simulink model "test_onoff_button_wrongpressionbehavior"  (R2022b)
settings: Solver=FixedStepAuto  StartTime=0.0  StopTime=240  FixedStep=0.1  RelTol=1e-3
settings Model: Creator=alewi  LastModifiedBy=cristian
settings ConfigComp: CovEnable=on  RecordCoverage=on  CovModelRefEnable=on

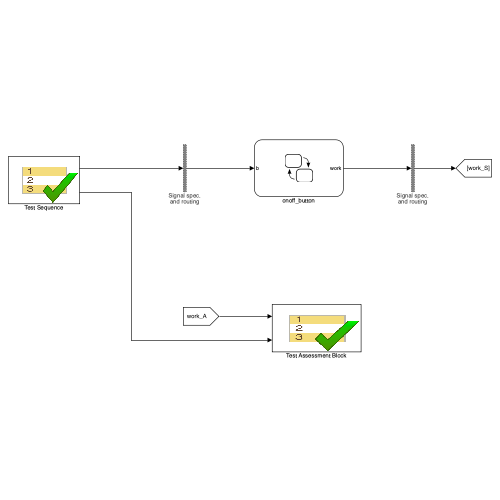
[thumbnail: Simulink's stored preview of the top-level diagram]
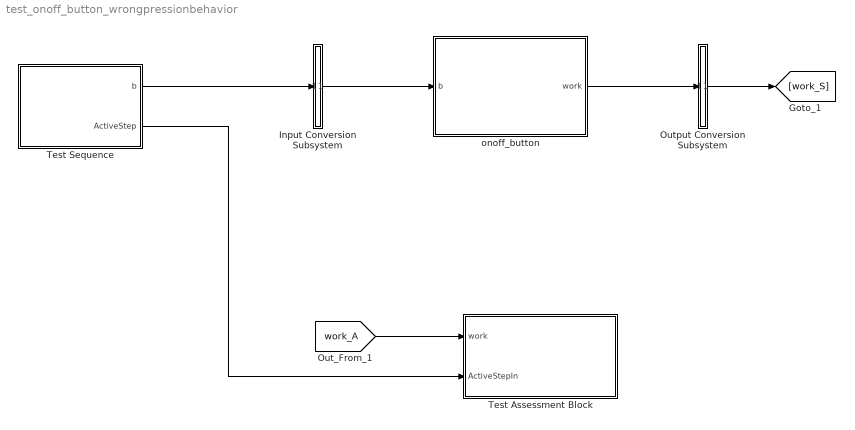
== system test_onoff_button_wrongpressionbehavior ==
  Input Conversion Subsystem : Subsystem  Tag=__SLT_ICS__  Description=|
      | Signal spec.
      | and routing
      settings: AttributesFormatString=%<Description>
  Output Conversion Subsystem : Subsystem  Tag=__SLT_OCS__  Description=|
      | Signal spec.
      | and routing
      settings: AttributesFormatString=%<Description>
  Test Assessment Block : Test Sequence  Tag=__SLT_ASMT__  TreatAsAtomicUnit=on
  Test Sequence : Test Sequence  TreatAsAtomicUnit=on
  onoff_button : Stateflow chart  TreatAsAtomicUnit=on
  wires:
  Output Conversion Subsystem/1(Outport_1) -> [work_S]
  Input Conversion Subsystem/1(Outport_1) -> onoff_button/1(b)
  onoff_button/1(work) -> Output Conversion Subsystem/1(Inport_1)
  Test Sequence/1(b) -> Input Conversion Subsystem/1(Inport_1)
  Test Sequence/2(ActiveStep) -> Test Assessment Block/2(ActiveStepIn)
  [work_A] -> Test Assessment Block/1(work)

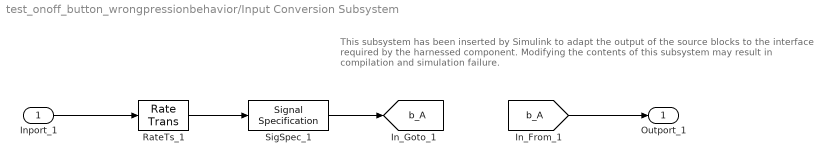
== system test_onoff_button_wrongpressionbehavior/Input Conversion Subsystem ==
  note: This subsystem has been inserted by Simulink to adapt the output of the source blocks to the interface required by the harnessed component.
      |  Modifying the contents of this subsystem may result in compilation and simulation failure.
  Inport_1 : Inport
  RateTs_1 : RateTransition  OutPortSampleTime=[-1, 0]
  SigSpec_1 : SignalSpecification  OutDataTypeStr=boolean  Dimensions=[1]  SampleTime=[-1, 0]
  Outport_1 : Outport
  tag scope: b_A=global
  wires:
  [b_A] -> Outport_1/1
  SigSpec_1/1 -> [b_A]
  RateTs_1/1 -> SigSpec_1/1
  Inport_1/1 -> RateTs_1/1

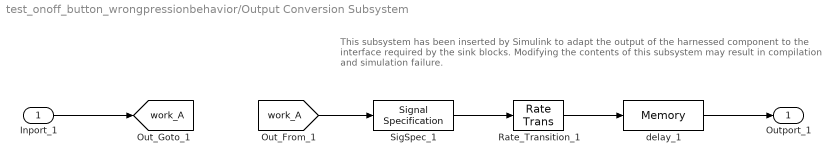
== system test_onoff_button_wrongpressionbehavior/Output Conversion Subsystem ==
  note: This subsystem has been inserted by Simulink to adapt the output of the harnessed component to the interface required by the sink blocks.
      |  Modifying the contents of this subsystem may result in compilation and simulation failure.
  Inport_1 : Inport
  Rate_Transition_1 : RateTransition  OutPortSampleTimeOpt=Inherit
  SigSpec_1 : SignalSpecification  OutDataTypeStr=boolean  Dimensions=[1]
  delay_1 : Memory
  Outport_1 : Outport
  tag scope: work_A=global
  wires:
  Inport_1/1 -> [work_A]
  [work_A] -> SigSpec_1/1
  SigSpec_1/1 -> Rate_Transition_1/1
  Rate_Transition_1/1 -> delay_1/1
  delay_1/1 -> Outport_1/1

== stateflow chart test_onoff_button_wrongpressionbehavior/Test Assessment Block ==
  state WrongPressionBehavior
    state Run
      state Verify_WB_Init
        verify(work == 0);
      state Verify_WB_Press
        verify(work == 1);
      state Verify_WB_Release
        verify(work == 1);
      state Verify_WB_LongPress
        verify(work == 1);
      state Verify_WB_Backto_Wait
        verify(work == 1);
      state Verify_LB_Void
      (default) -> (junction 404)
      Run -> (junction 404)
      (junction 404) -> (junction 405) [order 1] : [ActiveStepIn == ActiveStepEnumH2.WB_Init
          | ]
      (junction 405) -> Verify_WB_Init [order 1] : [~in(WrongPressionBehavior.Run.Verify_WB_Init)]
      (junction 404) -> (junction 413) [order 2]
      (junction 405) -> (junction 408) [order 2]
      (junction 413) -> (junction 414) [order 1] : [ActiveStepIn == ActiveStepEnumH2.WB_Press
          | ]
      (junction 414) -> Verify_WB_Press [order 1] : [~in(WrongPressionBehavior.Run.Verify_WB_Press)]
      (junction 413) -> (junction 421) [order 2]
      (junction 414) -> (junction 417) [order 2]
      (junction 421) -> (junction 422) [order 1] : [ActiveStepIn == ActiveStepEnumH2.WB_Release
          | ]
      (junction 422) -> Verify_WB_Release [order 1] : [~in(WrongPressionBehavior.Run.Verify_WB_Release)]
      (junction 421) -> (junction 429) [order 2]
      (junction 422) -> (junction 425) [order 2]
      (junction 429) -> (junction 430) [order 1] : [ActiveStepIn == ActiveStepEnumH2.WB_LongPress
          | ]
      (junction 430) -> Verify_WB_LongPress [order 1] : [~in(WrongPressionBehavior.Run.Verify_WB_LongPress)]
      (junction 429) -> (junction 437) [order 2]
      (junction 430) -> (junction 433) [order 2]
      (junction 437) -> (junction 438) [order 1] : [ActiveStepIn == ActiveStepEnumH2.WB_Backto_Wait
          | ]
      (junction 438) -> Verify_WB_Backto_Wait [order 1] : [~in(WrongPressionBehavior.Run.Verify_WB_Backto_Wait)]
      (junction 438) -> (junction 441) [order 2]
      (junction 446) -> (junction 447)
      (junction 447) -> Verify_LB_Void [order 1] : [~in(WrongPressionBehavior.Run.Verify_LB_Void)]
      (junction 447) -> (junction 450) [order 2]
      (junction 437) -> (junction 446) [order 2]
    (default) -> Run
  (default) -> WrongPressionBehavior : {assert(Active_Scenario_Index == 1,'The value of Scenario Parameter ''Active_Scenario_Index'' is not valid. Use the index of the scenario to specify it.')}
  data: work input boolean size=[1]; ActiveStepIn input; Active_Scenario_Index parameter =1

== stateflow chart test_onoff_button_wrongpressionbehavior/onoff_button ==
  note: Stato di accensione del bottone onoff
  note: In questo stato il bottone può accendere la macchina
  state INACTIVE
    state Pressed
      en: work = HIGH
    state Wait
      en: work = LOW
    (default) -> INACTIVE.Wait
    INACTIVE.Wait -> INACTIVE.Pressed : [b == PRESSED]
  note: Stato di spegnimento del bottone onoff
  note: In questo stato il bottone può spengere la macchina
  state ACTIVE
    state Wait
      en:
      b_long = RELEASED
    state Pressed
      en:
      b_long = RELEASED;
      on after(DURATION,sec): b_long = PRESSED
    state LongPressed
      en: work = LOW;
    (default) -> ACTIVE.Wait
    ACTIVE.Wait -> ACTIVE.Pressed : [b == PRESSED]
    ACTIVE.Pressed -> ACTIVE.Wait [order 1] : [b == RELEASED]
    ACTIVE.Pressed -> LongPressed [order 2] : [b_long == PRESSED && b == PRESSED]
  note: Se il bottone viene premuto una sola volta, il sistema viene acceso.
      | Se il bottone viene premuto per 1 secondo, il sistema viene spento.
      | Una pressione prolungata senza rilascio del bottone, non causa un alternarsi di accensioni e spegnimenti continui.
  (default) -> INACTIVE
  INACTIVE.Pressed -> ACTIVE : [b == RELEASED]
  LongPressed -> INACTIVE : [b==RELEASED]
  data: PRESSED constant boolean size=1 =0; RELEASED constant boolean size=1 =1; b input boolean size=1; DURATION constant double size=1 =1; b_long local boolean size=1; HIGH constant boolean size=1 =1; LOW constant boolean size=1 =0; work output boolean size=1

== stateflow chart test_onoff_button_wrongpressionbehavior/Test Sequence ==
  settings: updateMethod=DISCRETE  sampleTime=0.1
  state WrongPressionBehavior
    state WB_Init
      b = true
    state WB_Press
      b = false
      settings: description=|
          | Il bottone viene premuto per la prima volta.
          | L'output in questo caso è alto alla singola pressione.
          | Indipendentemente dal tempo in cui permango, non dovrei cambiare stato.
    state WB_Release
      b = true
      settings: description=|
          | Il bottone viene rilasciato.
          | Il sistema dovrebbe prepararsi al comportamento di un bottone a livelli, quindi cambia stato.
    state WB_LongPress
      b = false
      settings: description=Pressione prolungata ma troppo corta.
    state WB_Backto_Wait
      b = true
      settings: description=Rilascio definitivo.
    (default) -> WB_Init
    WB_Init -> WB_Press : [
        | true
        | ]
    WB_Press -> WB_Release : [
        | after(sample_time, sec)
        | ]
    WB_Release -> WB_LongPress : [
        | true
        | ]
    WB_LongPress -> WB_Backto_Wait : [
        | after(0.5, sec)
        | ]
  (default) -> WrongPressionBehavior : {assert(Active_Scenario_Index == 1,'The value of Scenario Parameter ''Active_Scenario_Index'' is not valid. Use the index of the scenario to specify it.')}
  data: b output boolean size=[1]; Active_Scenario_Index parameter =1; ActiveStep output Enum: ActiveStepEnumH2; sample_time constant double =str2num(get_param('InductionCooker','FixedStep'))
